simulink model "observing"  (R2025b)
settings: Solver=FixedStepDiscrete  StartTime=0.0  StopTime=Inf  FixedStep=0.01  RelTol=1e-3  EnableMultiTasking=on
undefined symbols (not defined in the file or in its folder): X, Y
libraries: MagLevTbx_BaseLib x5
settings Model: SimulationMode=external  ExtModeTrigDuration=2  Creator=riccardo  LastModifiedBy=miku
settings SolverCC: AutoInsertRateTranBlk=on
settings OptimizationCC: EnhancedBackFolding=on  PassReuseOutputArgsAs=Individual arguments  ZeroExternalMemoryAtStartup=off  ZeroInternalMemoryAtStartup=off  MaxStackSize=64  OptimizeBlockOrder=speed  DifferentSizesBufferReuse=on  OptimizationCustomize=off  EfficientTunableParamExpr=on
settings DebuggingCC: ParameterTunabilityLossMsg=error
settings HardwareCC: ProdBitPerPointer=32.0  ProdBitPerSizeT=32.0  ProdBitPerPtrDiffT=32.0  ProdLargestAtomicInteger=Long  ProdLargestAtomicFloat=Double  ProdWordSize=32.0  ProdHWDeviceType=ARM Compatible->ARM Cortex
settings SFSimCC: MATLABDynamicMemAlloc=off
settings RTWCC: SystemTargetFile=ert.tlc  HardwareBoard=Teensy 4.1 (Arduino Compatible)  TemplateMakefile=ert_default_tmf  Toolchain=Arduino ARM M7  BuildConfiguration=Faster Runs  Description=Embedded Coder
settings CodeAppCC: ForceParamTrailComments=on  IgnoreCustomStorageClasses=off  OperatorAnnotations=on  SimulinkDataObjDesc=on  SFDataObjDesc=on  InsertBlockDesc=on
settings ERTTargetCC: ExtModeTransport=3.0  ExtModeStaticAlloc=on  ExtModeAutomaticAllocSize=off  ExtModeStaticAllocSize=65536.0  ExtModeMexFile=ext_xcp  ExtModeIntrfLevel=Level2 - Open  InlinedParameterPlacement=Hierarchical  RootIOFormat=Structure reference  TargetLangStandard=C99 (ISO)  SupportContinuousTime=on  SupportVariableSizeSignals=on

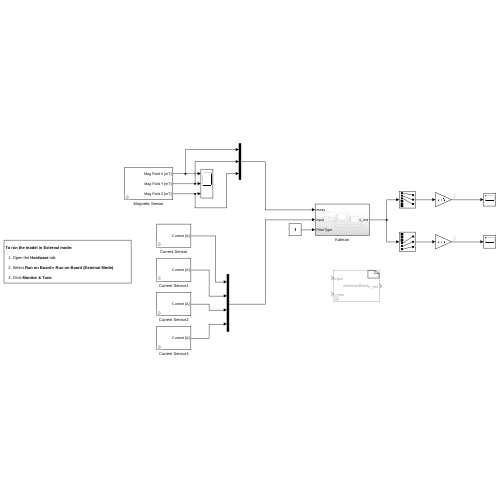
[thumbnail: Simulink's stored preview of the top-level diagram]
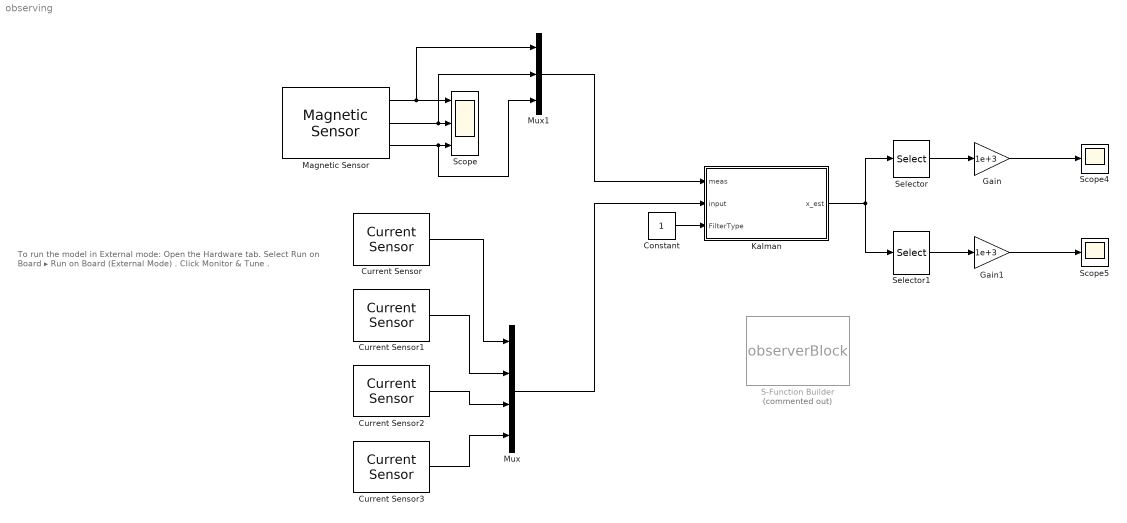
== system observing ==
  note: To run the model in External mode:
      | Open the Hardware tab.
      | Select Run on Board ▸ Run on Board (External Mode) .
      | Click Monitor & Tune .
  Constant : Constant
  Current Sensor : MagLevTbx_BaseLib/Inputs/Current Sensor  sensorId=+X  sampleTime=0.01  showEnablePort=off
      settings: SourceProductName=MagLev Toolbox
  Current Sensor1 : MagLevTbx_BaseLib/Inputs/Current Sensor  sensorId=-X  sampleTime=0.01  showEnablePort=off
      settings: SourceProductName=MagLev Toolbox
  Current Sensor2 : MagLevTbx_BaseLib/Inputs/Current Sensor  sensorId=+Y  sampleTime=0.01  showEnablePort=off
      settings: SourceProductName=MagLev Toolbox
  Current Sensor3 : MagLevTbx_BaseLib/Inputs/Current Sensor  sensorId=-Y  sampleTime=0.01  showEnablePort=off
      settings: SourceProductName=MagLev Toolbox
  Gain : Gain  Gain=1e+3
  Gain1 : Gain  Gain=1e+3
  Kalman : Subsystem
  Magnetic Sensor : MagLevTbx_BaseLib/Inputs/Magnetic Sensor  sensorId=Sensor 7  sampleTime=0.01  showEnablePort=off
      settings: SourceProductName=MagLev Toolbox
  Mux : Mux
  Mux1 : Mux  Inputs=3
  S-Function Builder : S-Function  Commented=on  FunctionName=observerBlock  SFunctionModules=observerBlock_wrapper.cpp matrices utilities observer  SFunctionDeploymentMode=off  EnableBusSupport=off  mask(S-Function Builder){}
      mask help: Simulink:masks:SFunctionBuilder_MD
      mask init:
      | val = [[.9  0.75 0.75 1 1 .9 .9 1]',[1 1 0.75 0.75 .9 .9 1 .9]'];try , sys = get_param(gcb,'SfunBuilderFcnName');if isempty(sys), sys = get_param(gcb,'FunctionName'); end,catch, sys = get_param(gcb,'FunctionName'); end
      settings: CopyFcn=set_param(gcbh,'LinkStatus','none')  OpenFcn=sfunctionwizard(gcbh)
      mask Display:
      | plot(val(:,1),val(:,2))
      | disp(sys)
      | port_label('input',1,sprintf('%s', 'input'),'interpreter','tex')
      | port_label('input',2,sprintf('%s', 'meas'),'interpreter','tex')
      | port_label('output',1,sprintf('%s', 'x\_est'),'interpreter','tex')
  Scope : Scope  NumInputPorts=3
      settings: ActiveDisplayYMinimum=-45.202162280701764  ActiveDisplayYMaximum=16.923712719298248
  Scope4 : Scope
      settings: ActiveDisplayYMinimum=-143.6458995161733  ActiveDisplayYMaximum=117.39550402407514  DataLoggingVariableName=ScopeData4
  Scope5 : Scope
      settings: ActiveDisplayYMinimum=-497.56216964625474  ActiveDisplayYMaximum=465.7377348762065  DataLoggingVariableName=ScopeData5
  Selector : Selector  InputPortWidth=6  IndexOptions=Index vector (dialog)  Indices=[1 2 3]  OutputSizes=1
  Selector1 : Selector  InputPortWidth=6  IndexOptions=Index vector (dialog)  Indices=[4 5 6]  OutputSizes=1
  wires:
  Magnetic Sensor/1 -> Mux1/1, Scope/1
  Magnetic Sensor/2 -> Mux1/2, Scope/2
  Magnetic Sensor/3 -> Mux1/3, Scope/3
  Current Sensor1/1 -> Mux/2
  Current Sensor/1 -> Mux/1
  Current Sensor3/1 -> Mux/4
  Current Sensor2/1 -> Mux/3
  Mux1/1 -> Kalman/1(meas)
  Mux/1 -> Kalman/2(input)
  Kalman/1(x_est) -> Selector1/1, Selector/1
  Selector/1 -> Gain/1
  Gain/1 -> Scope4/1
  Selector1/1 -> Gain1/1
  Gain1/1 -> Scope5/1
  Constant/1 -> Kalman/3(FilterType)

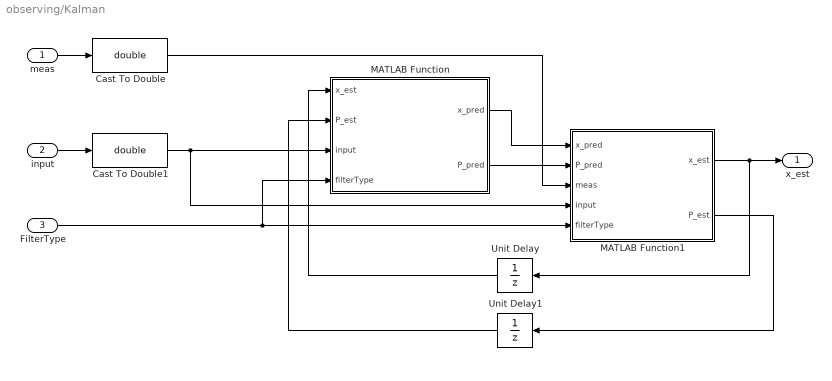
== system observing/Kalman ==
  meas : Inport
  input : Inport  Port=2
  FilterType : Inport  Port=3
  Cast To Double : DataTypeConversion  OutDataTypeStr=double  SaturateOnIntegerOverflow=off  RndMeth=Floor
  Cast To Double1 : DataTypeConversion  OutDataTypeStr=double  SaturateOnIntegerOverflow=off  RndMeth=Floor
  MATLAB Function : MATLAB Function  TreatAsAtomicUnit=on
  MATLAB Function1 : MATLAB Function  TreatAsAtomicUnit=on
  Unit Delay : UnitDelay  InitialCondition=zeros(6,1)  SampleTime=-1  HasFrameUpgradeWarning=on
  Unit Delay1 : UnitDelay  InitialCondition=eye(6,6)  SampleTime=-1  HasFrameUpgradeWarning=on
  x_est : Outport
  wires:
  MATLAB Function1/1(x_est) -> x_est/1, Unit Delay/1
  MATLAB Function1/2(P_est) -> Unit Delay1/1
  Unit Delay1/1 -> MATLAB Function/2(P_est)
  Unit Delay/1 -> MATLAB Function/1(x_est)
  meas/1 -> Cast To Double/1
  MATLAB Function/1(x_pred) -> MATLAB Function1/1(x_pred)
  MATLAB Function/2(P_pred) -> MATLAB Function1/2(P_pred)
  Cast To Double/1 -> MATLAB Function1/3(meas)
  input/1 -> Cast To Double1/1
  Cast To Double1/1 -> MATLAB Function/3(input), MATLAB Function1/4(input)
  FilterType/1 -> MATLAB Function1/5(filterType), MATLAB Function/4(filterType)

== matlab function observing/Kalman/MATLAB Function ==
  data: x_est input size=6; x_pred output double size=6; P_est input size=[6,6]; input input size=4; filterType input; P_pred output size=[6,6]; obs parameter

function [x_pred, P_pred] = Predict(x_est, P_est, input, filterType, obs)
    [x_pred_temp, P_pred_temp] = Prediction(x_est, P_est, input, filterType, obs);
    x_pred = x_pred_temp(1:6);
    P_pred = P_pred_temp(1:6, 1:6);
end

== matlab function observing/Kalman/MATLAB Function1 ==
  data: x_pred input size=6; x_est output double size=[6,1]; P_pred input size=[6,6]; meas input size=3; input input size=4; filterType input; P_est output size=[6,6]; obs parameter

function [x_est, P_est] = Update(x_pred, P_pred, meas, input, filterType, obs)
    [x_est_temp, P_est_temp] = Correction(x_pred, P_pred, meas, input, filterType, obs);
    x_est = x_est_temp(1:6);
    P_est = P_est_temp(1:6, 1:6);
end
